simulink model "VPC"  (R2021a)
settings: Solver=VariableStepAuto  StartTime=0.0  StopTime=50  FixedStep=0.001  RelTol=1e-3
model workspace (MAT data in the model file):
  lambda = 0.0016
  po = [0  0  0.5; 0.5  0  0; 0  0  -0.5; -0.5  0  0]
undefined symbols (not defined in the file or in its folder): mergepose
libraries: simlib_vpc_basic x4
settings Model: Creator=marco  LastModifiedBy=marco
settings SolverCC: AlgebraicLoopSolver=TrustRegion
settings DebuggingCC: AlgebraicLoopMsg=none  SFMachineParentedDataDiag=warning
settings RTWCC: Toolchain=Clang v3.1 | gmake (64-bit Mac)

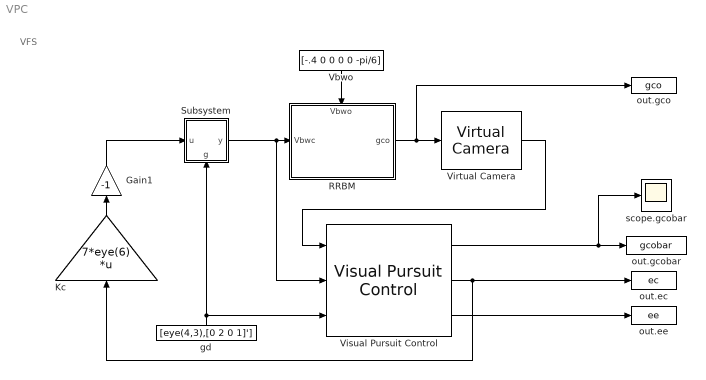
== system VPC ==
  note: VFS
  Gain1 : Gain  Gain=-1
  Kc : Gain  Gain=7*eye(6)  Multiplication=Matrix(K*u) (u vector)
  RRBM : Subsystem
      settings: PortSchema="{\"entries\":[{\"content\":{\"sides\":[{\"content\":{\"connectorIds\":[\"In1\"]},\"type\":\"ConnectorPlacement.EquallySpacedRectSide\",\"uuid\":\"ce1006a6-ff18-4db7-ad69-3a60144a672f\"},{\"content\":{\"connectorIds\":[\"Out1\"],\"side\":\"RIGHT\"},\"type\":\"ConnectorPlacement.EquallySpacedRectSide\",\"uuid\":\"9f6b7cf2-eb23-4db0-862a-f9244538bf77\"},{\"content\":{\"connectorIds\":[\"In2\"],\"side\":\"TOP\"},\"type\":\"ConnectorPlacement.EquallySpacedRectSide\",\"uuid\":\"e4abfdaf-0145-4439-9abb-46234dad4713\"},{\"content\":{\"connectorIds\":[],\"side\":\"HIDDEN\"},\"type\":\"ConnectorPlacement.EquallySpacedRectSide\",\"uuid\":\"77f0040d-d5e2-4b47-95e1-996605172696\"}]},\"type\":\"ConnectorPlacement.EquallySpacedConnector\",\"uuid\":\"a30e6cf8-5cfd-45cc-9c7f-0b16cc268ba1\"}],\"packageUris\":[\"http://schema.mathworks.com/mf0/Connector/R2020b\"],\"version\":\"1.0\"}"
      mask Display:
      | % Glitch in Matlab: If you define a line whose starting point and end point
      | % is equal, then the entire mask block is plotted in bold
      | plot([0,0],[0,0])
      | 
      | % Draw Box
      | plot([0,1,1,0,0],[0,0,1,1,0])
      | 
      | % Write label
      | fprintf('1 Agent\n1 Target','texmode','on')
      | 
      | % Label ports
      | port_label('input',1,'V^{b}_{wc}','texmode','on')
      | port_label('input',2,'V^{b}_{wo}','texmode','on')
      | port_label('output',1,'g_{co}','texmode','on')
  Subsystem : Subsystem
      settings: PortSchema="{\"entries\":[{\"content\":{\"sides\":[{\"content\":{\"connectorIds\":[\"In1\"]},\"type\":\"ConnectorPlacement.EquallySpacedRectSide\",\"uuid\":\"72e68008-5c4a-43a9-a560-64c6a31a0c08\"},{\"content\":{\"connectorIds\":[\"Out1\"],\"side\":\"RIGHT\"},\"type\":\"ConnectorPlacement.EquallySpacedRectSide\",\"uuid\":\"da07f5ff-2b2c-4c55-a2f2-34e133777503\"},{\"content\":{\"connectorIds\":[],\"side\":\"TOP\"},\"type\":\"ConnectorPlacement.EquallySpacedRectSide\",\"uuid\":\"6d174428-4364-4e89-aba7-4e9864808ab5\"},{\"content\":{\"connectorIds\":[\"In2\"],\"side\":\"BOTTOM\"},\"type\":\"ConnectorPlacement.EquallySpacedRectSide\",\"uuid\":\"f9633104-9c11-4d21-90a7-e0f886d9e92d\"},{\"content\":{\"connectorIds\":[],\"side\":\"HIDDEN\"},\"type\":\"ConnectorPlacement.EquallySpacedRectSide\",\"uuid\":\"662f08ae-9279-4a4f-85ea-81d97ead27d9\"}]},\"type\":\"ConnectorPlacement.EquallySpacedConnector\",\"uuid\":\"f3cd156c-cccd-47c6-b81c-6113f78efd58\"}],\"packageUris\":[\"http://schema.mathworks.com/mf0/Connector/R2020b\"],\"version\":\"1.0\"}"
      mask Display:
      | % Glitch in Matlab: If you define a line whose starting point and end point
      | % is equal, then the entire mask block is plotted in bold
      | plot([0,0],[0,0])
      | 
      | % Draw box
      | indent = 0.3;
      | ang=[0:0.2:pi/2, pi/2];
      | plot([0,1-indent],[0,0])
      | xp=indent*sin(ang)+1-indent;
      | yp=indent-indent*cos(ang);
      | plot(xp,yp);
      | plot([1,1,indent],[indent,1,1])
      | xp=indent-indent*sin(ang);
      | yp=1-indent+indent*cos(ang);
      | plot(xp,yp);
      | plot([0,0],[1-indent,0])
      | 
      | % Write label & ports
      | disp('-Ad_{(g_d)}','texmode','on')
      | text(0.5,0.2,'\fontsize{7}g_d','texmode','on')
  Vbwo : Constant  Value=[-.4 0 0 0 0 -pi/6]
  Virtual Camera : simlib_vpc_basic/Virtual Camera  camtype=Pinhole  po=po  lambda=lambda
      settings: SourceProductName=VPC Library
  Visual Pursuit Control : simlib_vpc_basic/Visual Pursuit Control  gd_source=external  gd_value=[eye(4,3),ones(4,1)]  show_ee=on  show_e=off  show_nu=off  show_dgcobar=off  show_gce=off  gcobar0=mergepose(eye(3),[0 1 0])  Ke_source=internal  Ke=15*eye(6)  show_ue_aux=off  projection=on  camtype=Pinhole  fo=po  lambda=lambda
      settings: SourceProductName=VPC Library
  gd : Constant  Value=[eye(4,3),[0 2 0 1]']
  out.ec : ToWorkspace  VariableName=ec  SaveFormat=Structure With Time  SampleTime=-1
  out.ee : ToWorkspace  VariableName=ee  SaveFormat=Structure With Time  SampleTime=-1
  out.gco : ToWorkspace  VariableName=gco  SaveFormat=Structure With Time  SampleTime=-1
  out.gcobar : ToWorkspace  VariableName=gcobar  SaveFormat=Structure With Time  SampleTime=-1
  scope.gcobar : Scope
  wires:
  Vbwo/1 -> RRBM/2(Vbwo)
  RRBM/1(gco) -> Virtual Camera/1, out.gco/1
  Virtual Camera/1 -> Visual Pursuit Control/1
  Visual Pursuit Control/1 -> scope.gcobar/1, out.gcobar/1
  Kc/1 -> Gain1/1
  Visual Pursuit Control/2 -> Kc/1, out.ec/1
  Visual Pursuit Control/3 -> out.ee/1
  Subsystem/1(y) -> Visual Pursuit Control/2, RRBM/1(Vbwc)
  Gain1/1 -> Subsystem/1(u)
  gd/1 -> Subsystem/2(g), Visual Pursuit Control/3

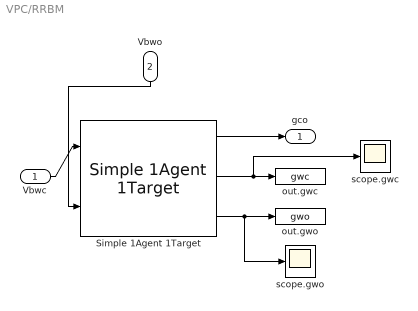
== system VPC/RRBM ==
  Vbwc : Inport
  Vbwo : Inport  Port=2
  Simple 1Agent 1Target : simlib_vpc_basic/Simple 1Agent 1Target  gwc0=mergepose(eye(3),[0 -5 0])  projectionAgent=on  gwo0=mergepose(eye(3),[0.3 0.1 0.1])  projectionTarget=on  showgwc=on  showdgwc=off  showgwo=on  showdgwo=off
      settings: SourceProductName=VPC Library
  out.gwc : ToWorkspace  VariableName=gwc  SaveFormat=Structure With Time  SampleTime=-1
  out.gwo : ToWorkspace  VariableName=gwo  SaveFormat=Structure With Time  SampleTime=-1
  scope.gwc : Scope
  scope.gwo : Scope
  gco : Outport
  wires:
  Vbwo/1 -> Simple 1Agent 1Target/2
  Vbwc/1 -> Simple 1Agent 1Target/1
  Simple 1Agent 1Target/1 -> gco/1
  Simple 1Agent 1Target/2 -> scope.gwc/1, out.gwc/1
  Simple 1Agent 1Target/3 -> scope.gwo/1, out.gwo/1

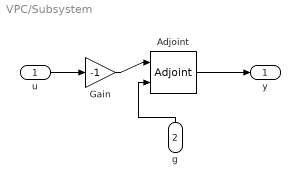
== system VPC/Subsystem ==
  u : Inport
  g : Inport  Port=2
  Adjoint : simlib_vpc_basic/Adjoint  adjointtype=pose
      settings: SourceProductName=VPC Library
  Gain : Gain  Gain=-1
  y : Outport
  wires:
  Adjoint/1 -> y/1
  u/1 -> Gain/1
  g/1 -> Adjoint/2
  Gain/1 -> Adjoint/1
